simulink model "singlephase"  (R2015b)
settings: Solver=VariableStepAuto  StartTime=0.0  StopTime=1  RelTol=1e-3
undefined symbols (not defined in the file): Ts, w1
libraries: simulink x1, powerlib x1
settings Model: Creator=HP  LastModifiedBy=HP

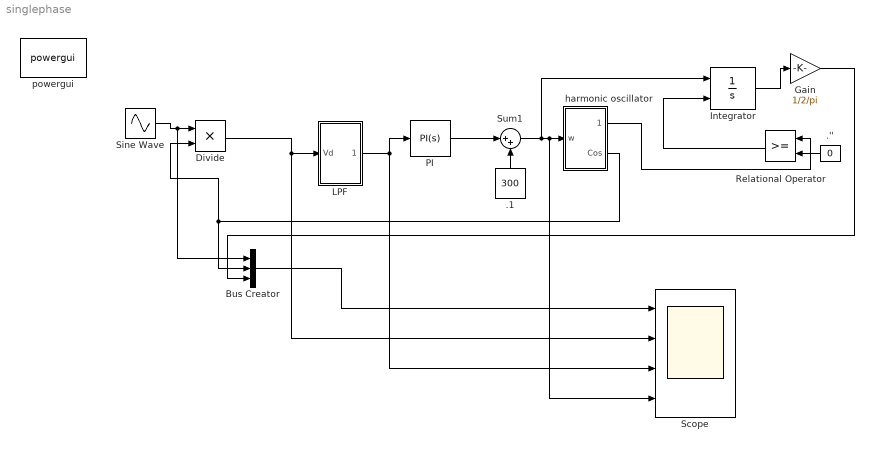
== system singlephase ==
  .'' : Constant  Value=0
  .1 : Constant  Value=300
  Bus Creator : BusCreator  Inputs=3
  Divide : Product
  Gain : Gain  Gain=1/2/pi
  Integrator : Integrator  ExternalReset=rising  UpperSaturationLimit=2*pi  LowerSaturationLimit=0
  LPF : Subsystem
  PI : simulink/Continuous/PID Controller  Controller=PI  TimeDomain=Continuous-time  SampleTime=-1  IntegratorMethod=Forward Euler  FilterMethod=Forward Euler  Form=Parallel  UseFilter=on  ControllerParametersSource=internal  P=50  I=320  D=0  N=100  InitialConditionSource=internal  InitialConditionForIntegrator=0  InitialConditionForFilter=0  ExternalReset=none  ZeroCross=off  LimitOutput=off  UpperSaturationLimit=inf  LowerSaturationLimit=-inf  LinearizeAsGain=on  AntiWindupMode=none  Kb=1  TrackingMode=off  Kt=1  PParamMin=[]  PParamMax=[]  IParamMin=[]  IParamMax=[]  DParamMin=[]  DParamMax=[]  NParamMin=[]  NParamMax=[]  KbParamMin=[]  KbParamMax=[]  KtParamMin=[]  KtParamMax=[]  POutMin=[]  POutMax=[]  IOutMin=[]  IOutMax=[]  DOutMin=[]  DOutMax=[]  NOutMin=[]  NOutMax=[]  KbOutMin=[]  KbOutMax=[]  KtOutMin=[]  KtOutMax=[]  IntegratorOutMin=[]  IntegratorOutMax=[]  FilterOutMin=[]  FilterOutMax=[]  SumOutMin=[]  SumOutMax=[]  SumI1OutMin=[]  SumI1OutMax=[]  SumI2OutMin=[]  SumI2OutMax=[]  SumI3OutMin=[]  SumI3OutMax=[]  SumDOutMin=[]  SumDOutMax=[]  SaturationOutMin=[]  SaturationOutMax=[]  IntegratorContinuousStateAttributes=''  IntegratorStateMustResolveToSignalObject=off  IntegratorRTWStateStorageClass=Auto  FilterContinuousStateAttributes=''  FilterStateMustResolveToSignalObject=off  FilterRTWStateStorageClass=Auto  DifferentiatorICPrevScaledInput=0  DifferentiatorOutMin=[]  DifferentiatorOutMax=[]
  Relational Operator : RelationalOperator  OutDataTypeStr=boolean
  Scope : Scope  NumInputPorts=4
  Sine Wave : Sin  Frequency=w1  SampleTime=Ts
  Sum1 : Sum  Inputs=|++
  "harmonic oscillator " : Subsystem
  powergui : powerlib/powergui  Priority=1  SimulationMode=Continuous  SolverType=Tustin/Backward Euler (TBE)  SampleTime=50e-6  frequency=60  SPID=on  DisableSnubberDevices=off  DisableRonSwitches=off  DisableVfSwitches=off  SwTol=0  DisplayEquations=on  Interpol=off  ExternalGateDelay=off  methode=off  Ts=10  FunctionMessages=off  echomessages=off  HookPort=off  EnableUseOfTLC=off  x0status=blocks  frequencyindice=50  Pbase=100e6  ErrMax=1e-4  Iterations=50  UnitsV=kV  UnitsW=MW  buscounter=0  RestoreLinks=warning  ResistiveCurrentMeasurement=off  Frange=[0:2:500]  Ylog=off  Xlog=on  ShowGrid=off  save=off  variable=ZData  structure=Vload  ZoomFFT=on  StartTime=0.2  cycles=4  DisplayStyle=3  fundamental=50  FreqAxis=on  MaxFrequency=1000  frequencyindicesteady=1  RmsSteady=1  display=off
  wires:
  Sine Wave/1 -> Bus Creator/1, Divide/1
  "harmonic oscillator "/2(Cos) -> Divide/2, Bus Creator/2
  .1/1 -> Sum1/2
  PI/1 -> Sum1/1
  Divide/1 -> Scope/2, LPF/1(Vd)
  "harmonic oscillator "/1(Sine) -> Relational Operator/1
  .''/1 -> Relational Operator/2
  Sum1/1 -> Scope/4, "harmonic oscillator "/1(w), Integrator/1
  Relational Operator/1 -> Integrator/2
  Bus Creator/1 -> Scope/1
  Integrator/1 -> Gain/1
  Gain/1 -> Bus Creator/3
  LPF/1(Vde) -> PI/1, Scope/3

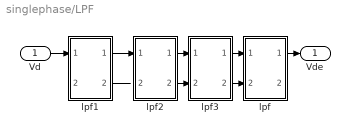
== system singlephase/LPF ==
  Vd : Inport
  lpf : Subsystem
  lpf1 : Subsystem
  lpf2 : Subsystem
  lpf3 : Subsystem
  Vde : Outport
  wires:
  lpf1/2(Out2) -> ?
  ? -> ?
  ? -> lpf1/2(In2)
  Vd/1 -> lpf1/1(In1)
  lpf2/2(Out2) -> lpf3/2(In2)
  lpf2/1(Out1) -> lpf3/1(In1)
  lpf3/1(Out1) -> lpf/1(In1)
  lpf3/2(Out2) -> lpf/2(In2)
  lpf1/1(Out1) -> lpf2/1(In1)
  lpf/1(Out1) -> Vde/1

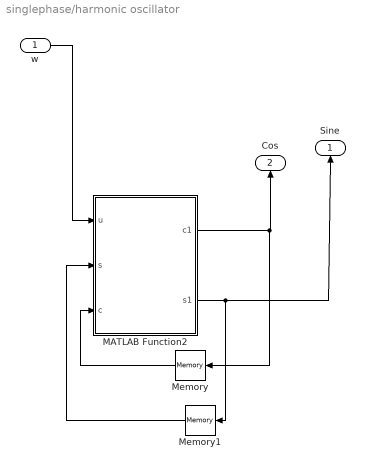
== system singlephase/harmonic oscillator  ==
  w : Inport
  MATLAB Function2 : MATLAB Function  TreatAsAtomicUnit=on
  Memory : Memory  X0=1
  Memory1 : Memory
  Sine : Outport
  Cos : Outport  Port=2
  wires:
  Memory1/1 -> MATLAB Function2/2(s)
  MATLAB Function2/2(s1) -> Sine/1, Memory1/1
  MATLAB Function2/1(c1) -> Cos/1, Memory/1
  Memory/1 -> MATLAB Function2/3(c)
  w/1 -> MATLAB Function2/1(u)

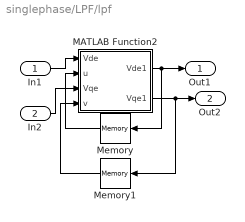
== system singlephase/LPF/lpf ==
  In1 : Inport
  In2 : Inport  Port=2
  MATLAB Function2 : MATLAB Function  TreatAsAtomicUnit=on
  Memory : Memory
  Memory1 : Memory
  Out1 : Outport
  Out2 : Outport  Port=2
  wires:
  MATLAB Function2/1(Vde1) -> Out1/1, Memory/1
  In1/1 -> MATLAB Function2/1(Vde)
  Memory/1 -> MATLAB Function2/2(u)
  In2/1 -> MATLAB Function2/3(Vqe)
  MATLAB Function2/2(Vqe1) -> Out2/1, Memory1/1
  Memory1/1 -> MATLAB Function2/4(v)

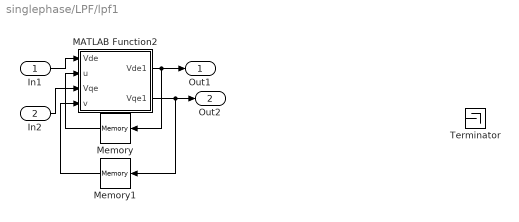
== system singlephase/LPF/lpf1 ==
  In1 : Inport
  In2 : Inport  Port=2
  MATLAB Function2 : MATLAB Function  TreatAsAtomicUnit=on
  Memory : Memory
  Memory1 : Memory
  Terminator : Terminator
  Out1 : Outport
  Out2 : Outport  Port=2
  wires:
  MATLAB Function2/1(Vde1) -> Out1/1, Memory/1
  In1/1 -> MATLAB Function2/1(Vde)
  Memory/1 -> MATLAB Function2/2(u)
  In2/1 -> MATLAB Function2/3(Vqe)
  MATLAB Function2/2(Vqe1) -> Out2/1, Memory1/1
  Memory1/1 -> MATLAB Function2/4(v)

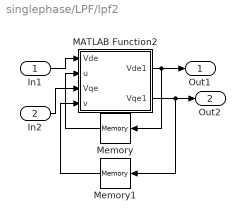
== system singlephase/LPF/lpf2 ==
  In1 : Inport
  In2 : Inport  Port=2
  MATLAB Function2 : MATLAB Function  TreatAsAtomicUnit=on
  Memory : Memory
  Memory1 : Memory
  Out1 : Outport
  Out2 : Outport  Port=2
  wires:
  MATLAB Function2/1(Vde1) -> Out1/1, Memory/1
  In1/1 -> MATLAB Function2/1(Vde)
  Memory/1 -> MATLAB Function2/2(u)
  In2/1 -> MATLAB Function2/3(Vqe)
  MATLAB Function2/2(Vqe1) -> Out2/1, Memory1/1
  Memory1/1 -> MATLAB Function2/4(v)

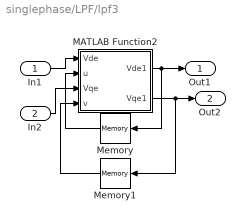
== system singlephase/LPF/lpf3 ==
  In1 : Inport
  In2 : Inport  Port=2
  MATLAB Function2 : MATLAB Function  TreatAsAtomicUnit=on
  Memory : Memory
  Memory1 : Memory
  Out1 : Outport
  Out2 : Outport  Port=2
  wires:
  MATLAB Function2/1(Vde1) -> Out1/1, Memory/1
  In1/1 -> MATLAB Function2/1(Vde)
  Memory/1 -> MATLAB Function2/2(u)
  In2/1 -> MATLAB Function2/3(Vqe)
  MATLAB Function2/2(Vqe1) -> Out2/1, Memory1/1
  Memory1/1 -> MATLAB Function2/4(v)

== matlab function singlephase/LPF/lpf1/MATLAB Function2 ==
  data: Vde input; Vde1 output; u input; Vqe input; v input; Vqe1 output
function [Vde1,Vqe1] = fcn(Vde,u,Vqe,v)
%#codegen
Ts=5e-5;
a=Ts/0.009;
%Vde1=u*a/(a+1)+(1/(1+a))*(Vde-u);
%Vqe1=v*a/(a+1)+(1/(1+a))*(Vqe-v);
Vde1=u+a*(Vde-u);
Vqe1=v+a*(Vqe-v);
end

== matlab function singlephase/LPF/lpf2/MATLAB Function2 ==
  data: Vde input; Vde1 output; u input; Vqe input; v input; Vqe1 output
function [Vde1,Vqe1] = fcn(Vde,u,Vqe,v)
%#codegen
Ts=5e-5;
a=Ts/0.009;
%Vde1=u*a/(a+1)+(1/(1+a))*(Vde-u);
%Vqe1=v*a/(a+1)+(1/(1+a))*(Vqe-v);
Vde1=u+a*(Vde-u);
Vqe1=v+a*(Vqe-v);
end

== matlab function singlephase/harmonic oscillator /MATLAB Function2 ==
  data: u input; s input; c input; c1 output; s1 output
function [c1,s1] = fcn(u,s,c)

Ts=5e-5;

    s1=s+u*Ts*c;
    
    c1=c-u*Ts*s1;
    if c1>1
        s1=0;
        c1=1;

    end
        
    
%     i1=i+0.001;
%     if >0.42
%        i=0;i1=0;
%         c1=1;
%         s1=0;
%     end

== matlab function singlephase/LPF/lpf/MATLAB Function2 ==
  data: Vde input; Vde1 output; u input; Vqe input; v input; Vqe1 output
function [Vde1,Vqe1] = fcn(Vde,u,Vqe,v)
%#codegen
Ts=5e-5;
a=Ts/0.009;
%Vde1=u*a/(a+1)+(1/(1+a))*(Vde-u);
%Vqe1=v*a/(a+1)+(1/(1+a))*(Vqe-v);
Vde1=u+a*(Vde-u);
Vqe1=v+a*(Vqe-v);
end

== matlab function singlephase/LPF/lpf3/MATLAB Function2 ==
  data: Vde input; Vde1 output; u input; Vqe input; v input; Vqe1 output
function [Vde1,Vqe1] = fcn(Vde,u,Vqe,v)
%#codegen
Ts=5e-5;
a=Ts/0.009;
%Vde1=u*a/(a+1)+(1/(1+a))*(Vde-u);
%Vqe1=v*a/(a+1)+(1/(1+a))*(Vqe-v);
Vde1=u+a*(Vde-u);
Vqe1=v+a*(Vqe-v);
end
